simulink model "servo1"  (Simulink 6.5)
settings: Solver=ode23s  StartTime=0.0  StopTime=10.0  RelTol=1e-3
values from neighbouring files (symbols this model uses):
  sin_dist_amp = 1    [macro.m]
  sin_dist_freq = 100*pi    (= 314.159265359)    [macro.m]
  step_size = 0    [macro.m]
  u_max = inf    [macro.m]
  white_noise_var = 0    [macro.m]
libraries: cstblocks x2, simulink x1
settings Model: Creator=Marcus  LastModifiedBy=Administrat?r
settings DebuggingCC: SignalResolutionControl=UseLocalSettings

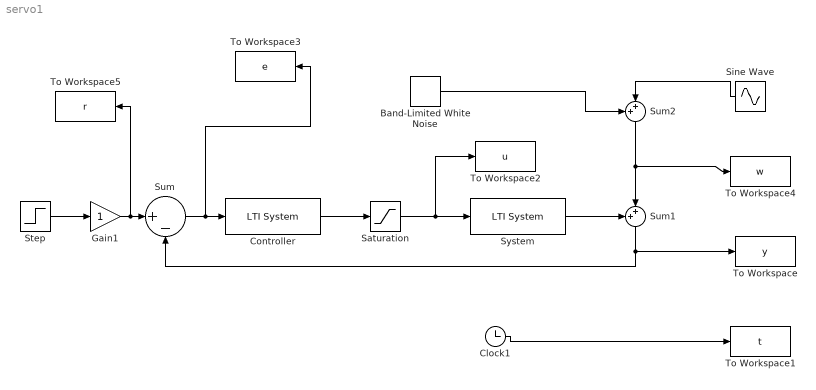
== system servo1 ==
  Band-Limited White Noise : simulink/Sources/Band-Limited White Noise  SystemSampleTime=-1  Cov=[white_noise_var]  Ts=0.1  seed=[23341]
  Clock1 : Clock
      settings: Decimation=10
  Controller : cstblocks/LTI System  SystemSampleTime=-1  sys=Fsim  IC=[]
  Gain1 : Gain
  Saturation : Saturate  UpperLimit=u_max  LowerLimit=-u_max
  Sine Wave : Sin  Orientation=left  Amplitude=sin_dist_amp  Frequency=sin_dist_freq  SampleTime=0
  Step : Step  After=step_size  SampleTime=0
  Sum : Sum  Inputs=|+-
  Sum1 : Sum  Orientation=down  Inputs=++|
  Sum2 : Sum  Orientation=down  Inputs=++|
  System : cstblocks/LTI System  SystemSampleTime=-1  sys=Gsim  IC=[]
  To Workspace : ToWorkspace  VariableName=y  SampleTime=-1  SaveFormat=Array
  To Workspace1 : ToWorkspace  VariableName=t  SampleTime=-1  SaveFormat=Array
  To Workspace2 : ToWorkspace  VariableName=u  SampleTime=-1  SaveFormat=Array
  To Workspace3 : ToWorkspace  VariableName=e  SampleTime=-1  SaveFormat=Array
  To Workspace4 : ToWorkspace  VariableName=w  SampleTime=-1  SaveFormat=Array
  To Workspace5 : ToWorkspace  VariableName=r  SampleTime=-1  SaveFormat=Array
  wires:
  Clock1/1 -> To Workspace1/1
  System/1 -> Sum1/1
  Sum1/1 -> Sum/2, To Workspace/1
  Controller/1 -> Saturation/1
  Saturation/1 -> System/1, To Workspace2/1
  Gain1/1 -> Sum/1, To Workspace5/1
  Step/1 -> Gain1/1
  Sum/1 -> Controller/1, To Workspace3/1
  Band-Limited White Noise/1 -> Sum2/1
  Sine Wave/1 -> Sum2/2
  Sum2/1 -> Sum1/2, To Workspace4/1
